simulink model "motorsim"  (R2021a)
settings: Solver=VariableStepAuto  StartTime=0.0  StopTime=10  RelTol=1e-3
values from neighbouring files (symbols this model uses):
  Ts = 1.0/20    (= 0.05)    [motorcodelast.m]
undefined symbols (not defined in the file or in its folder): DiscIntNeverNeededParam
libraries: simulink x5, rllib x1
settings Model: Creator=User  LastModifiedBy=User

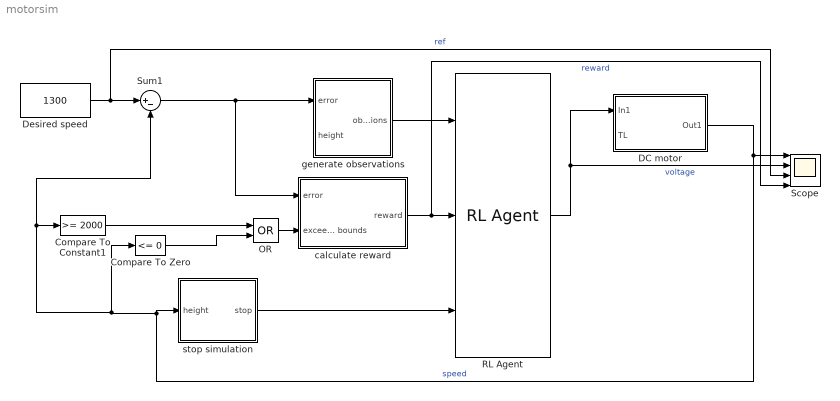
== system motorsim ==
  Compare To Constant1 : simulink/Logic and Bit Operations/Compare To Constant  relop=>=  const=2000  OutDataTypeStr=boolean
  Compare To Zero : simulink/Logic and Bit Operations/Compare To Zero  relop=<=  OutDataTypeStr=boolean
  DC motor : Subsystem  mask{Ra=1, La=0.5, J=0.01, D=0.1}
      mask prompts: Ra "Armature Resistance (Ra)"; La "Armature Inductance (La)"; J "Inertia (J)"; D "Damping (B)"
  Desired speed : Constant  Value=1300
  OR : Logic  Operator=OR  IconShape=distinctive  AllPortsSameDT=off  OutDataTypeStr=boolean
  RL Agent : rllib/RL Agent  Agent=agent  ExternalActionAsInput=off  ProvideCumRwd=off  TreatAsDirectFeedthrough=on
  Scope : Scope  NumInputPorts=4
  Sum1 : Sum  Inputs=|+-  SaturateOnIntegerOverflow=on
  calculate reward : Subsystem
  generate observations : Subsystem
  stop simulation : Subsystem
  wires:
  OR/1 -> calculate reward/2(exceeds bounds)
  Compare To Constant1/1 -> OR/1
  Compare To Zero/1 -> OR/2
  RL Agent/1 -> DC motor/1(In1), Scope/2  "voltage"
  generate observations/1(observations) -> RL Agent/1
  stop simulation/1(stop) -> RL Agent/3
  Sum1/1 -> calculate reward/1(error), generate observations/1(error)
  calculate reward/1(reward) -> Scope/4, RL Agent/2  "reward"
  Desired speed/1 -> Scope/3, Sum1/1  "ref"
  DC motor/1(Out1) -> Sum1/2, Compare To Constant1/1, Compare To Zero/1, stop simulation/1(height), Scope/1  "speed"

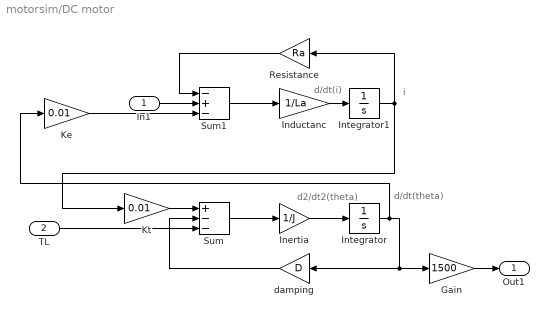
== system motorsim/DC motor ==
  note: d/dt(i)
  note: i
  note: d/dt(theta)
  note: d2/dt2(theta)
  In1 : Inport
  TL : Inport  Port=2
  Gain : Gain  Gain=1500
  Inductanc : Gain  Gain=1/La  SaturateOnIntegerOverflow=on  OutDataTypeStr=Inherit: Same as input  ParamDataTypeStr=Inherit: Same as input
  Inertia : Gain  Gain=1/J  SaturateOnIntegerOverflow=on  OutDataTypeStr=Inherit: Same as input  ParamDataTypeStr=Inherit: Same as input
  Integrator : Integrator
  Integrator1 : Integrator
  Ke : Gain  Gain=0.01  SaturateOnIntegerOverflow=on  OutDataTypeStr=Inherit: Same as input  ParamDataTypeStr=Inherit: Same as input
  Kt : Gain  Gain=0.01  SaturateOnIntegerOverflow=on  OutDataTypeStr=Inherit: Same as input  ParamDataTypeStr=Inherit: Same as input
  Resistance : Gain  Gain=Ra  SaturateOnIntegerOverflow=on  OutDataTypeStr=Inherit: Same as input  ParamDataTypeStr=Inherit: Same as input
  Sum : Sum  Inputs=+--  InputSameDT=on  SaturateOnIntegerOverflow=on  OutDataTypeStr=Inherit: Same as first input
  Sum1 : Sum  Inputs=-+-  InputSameDT=on  SaturateOnIntegerOverflow=on  OutDataTypeStr=Inherit: Same as first input
  damping : Gain  Gain=D  SaturateOnIntegerOverflow=on  OutDataTypeStr=Inherit: Same as input  ParamDataTypeStr=Inherit: Same as input
  Out1 : Outport
  wires:
  Integrator1/1 -> Resistance/1, Kt/1
  Integrator/1 -> Ke/1, Gain/1, damping/1
  Ke/1 -> Sum1/3
  Resistance/1 -> Sum1/1
  Kt/1 -> Sum/1
  damping/1 -> Sum/2
  Sum1/1 -> Inductanc/1
  Sum/1 -> Inertia/1
  Inertia/1 -> Integrator/1
  Inductanc/1 -> Integrator1/1
  In1/1 -> Sum1/2
  TL/1 -> Sum/3
  Gain/1 -> Out1/1

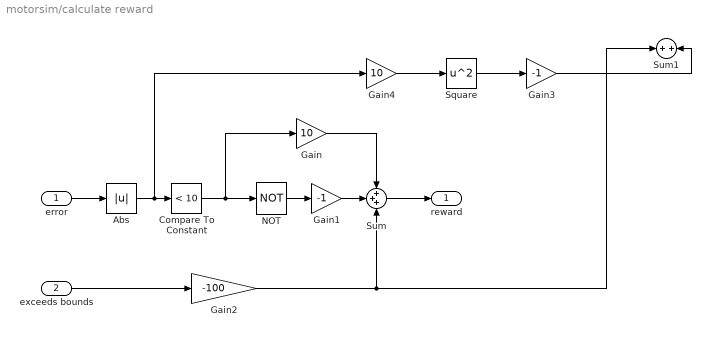
== system motorsim/calculate reward ==
  error : Inport
  exceeds bounds : Inport  Port=2
  Abs : Abs
  Compare To Constant : simulink/Logic and Bit Operations/Compare To Constant  relop=<  const=10  OutDataTypeStr=boolean
  Gain : Gain  Gain=10
  Gain1 : Gain  Gain=-1
  Gain2 : Gain  Gain=-100
  Gain3 : Gain  Gain=-1
  Gain4 : Gain  Gain=10
  NOT : Logic  Operator=NOT  IconShape=distinctive  AllPortsSameDT=off  OutDataTypeStr=boolean
  Square : Math  Operator=square  SaturateOnIntegerOverflow=on
  Sum : Sum  Inputs=+++  OutDataTypeStr=double
  Sum1 : Sum  OutDataTypeStr=double
  reward : Outport  VectorParamsAs1DForOutWhenUnconnected=off
  wires:
  Gain2/1 -> Sum1/1, Sum/3
  Gain/1 -> Sum/1
  Compare To Constant/1 -> NOT/1, Gain/1
  Gain1/1 -> Sum/2
  NOT/1 -> Gain1/1
  exceeds bounds/1 -> Gain2/1
  error/1 -> Abs/1
  Gain3/1 -> Sum1/2
  Abs/1 -> Compare To Constant/1, Gain4/1
  Gain4/1 -> Square/1
  Square/1 -> Gain3/1
  Sum/1 -> reward/1

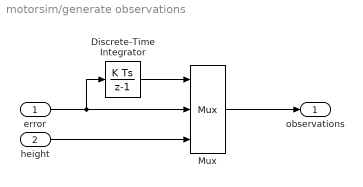
== system motorsim/generate observations ==
  error : Inport
  height : Inport  Port=2
  Discrete-Time Integrator : DiscreteIntegrator  SampleTime=Ts  ICPrevOutput=DiscIntNeverNeededParam  ICPrevScaledInput=DiscIntNeverNeededParam
  Mux : Mux  Inputs=3
  observations : Outport  VectorParamsAs1DForOutWhenUnconnected=off
  wires:
  height/1 -> Mux/3
  Discrete-Time Integrator/1 -> Mux/1
  error/1 -> Discrete-Time Integrator/1, Mux/2
  Mux/1 -> observations/1

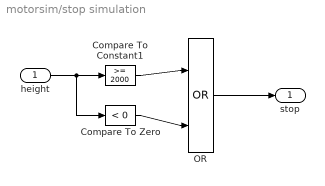
== system motorsim/stop simulation ==
  height : Inport
  Compare To Constant1 : simulink/Logic and Bit Operations/Compare To Constant  relop=>=  const=2000  OutDataTypeStr=boolean
  Compare To Zero : simulink/Logic and Bit Operations/Compare To Zero  relop=<  OutDataTypeStr=boolean
  OR : Logic  Operator=OR  IconShape=distinctive  AllPortsSameDT=off  OutDataTypeStr=boolean
  stop : Outport  VectorParamsAs1DForOutWhenUnconnected=off
  wires:
  height/1 -> Compare To Zero/1, Compare To Constant1/1
  Compare To Zero/1 -> OR/2
  Compare To Constant1/1 -> OR/1
  OR/1 -> stop/1
